simulink model "bh_compare_hand_MCKG_to_Ab"  (R2020b)
settings: Solver=ode23t  StartTime=0.0  StopTime=50  FixedStep=0.001  RelTol=1e-5  EnableMultiTasking=on
values from neighbouring files (symbols this model uses):
  K = [0.0865712753524 0.00277244570809 -0.0192153083791 -0.00162453351485 3.32348361895e-08 -1.41900444311e-08 -0.0932413563659 2.38058592401e-06 6.56188614095e-09 -0.0932413743514 2.52459639721e-09 9.53911962763e-08 ... (84 elements, 4x21)]    [CONFIRMED_bh_CONT_DES_RESULTS.mat]    (also in CONFIRMED_bh_CONT_DES_RESULTS_DISCRETE.mat = [-4.44584196463e-19 1.60298866655e-18 6.22915677006e-18 0 -9; CONFIRMED_bh_CONT_DES_RESULTS_DISCRETE_PRE_19a_using_DARE_SOLVER.mat = [-0.000193022438438 0.000285510081841 0.000531074046333 0.00; CONFIRMED_bh_CONT_DES_RESULTS_DISCRETE_R2019b.mat = [3.0073494701e-20 1.31173839205e-18 -5.80308139081e-19 0 8.7; CONFIRMED_bh_CONT_DES_RESULTS_PRE_19a_using_CARE_SOLVER.mat = [3.8473936011e-07 5.10337913269e-05 5.50269068807e-05 0.0072)
undefined symbols (not defined in the file or in its folder): P_elec, P_mot, P_one_prop, P_pend, P_veh, sigbuilder_block
libraries: simulink_extras x42, bh_6dof_LIBRARY x42, pid_lib x8, simulink x6
(part 1 of 3)
settings Model: Creator=bhorton  LastModifiedBy=bhorton
settings SolverCC: ZeroCrossAlgorithm=Adaptive
settings DataIOCC: SaveOutput=off  SignalLogging=off  DSMLogging=off  VisualizeSimOutput=off  SaveTime=off  ReturnWorkspaceOutputs=off
settings OptimizationCC: LifeSpan=inf
settings DebuggingCC: AllowSymbolicDim=off  PregeneratedLibrarySubsystemCodeDiagnostic=none  SFUnexpectedBacktrackingDiag=warning  SFNoUnconditionalDefaultTransitionDiag=warning  SFExecutionAtInitializationDiag=none  ArithmeticOperatorsInVariantConditions=warning
settings ModelReferenceCC: PropagateSignalLabelsOutOfModel=off
settings SFSimCC: SimUseLocalCustomCode=off  CustomCodeUndefinedFunction=UseInterfaceOnly
settings RTWCC: RTWUseLocalCustomCode=off
settings CodeAppCC: StateflowObjectComments=on
settings GRTTargetCC: TargetLangStandard=C89/C90 (ANSI)
settings ConfigComp: CovMetricSettings=dw  CovSaveCumulativeToWorkspaceVar=on  CovSaveSingleToWorkspaceVar=on  CovExternalEMLEnable=off
settings SimscapeCC: SimscapeNormalizeSystem=off
settings ExplorerConfigSet: InternalSimMechanicsExplorerSettings="<ExplorerConfiguration><canonicalview>default</canonicalview><AnimationSetting><BasePlaybackSpeed>1.0</BasePlaybackSpeed><PlaybackSpeedFactor>1.0</PlaybackSpeedFactor></AnimationSetting><TilePanel><TileInfo><Tiles Columns=\"2\" Count=\"4\" Rows=\"2\"><Column Weight=\"0.5\"/><Column Weight=\"0.5\"/><Row Weight=\"0.4994\"/><Row Weight=\"0.5006\"/><Tile Height=\"1\" Width=\"1\" X=\"0\" Y=\"0\"/><Tile Height=\"1\" Width=\"1\" X=\"0\" Y=\"1\"/><Tile Height=\"1\" Width=\"1\" X=\"1\" Y=\"0\"/><Tile Height=\"1\" Width=\"1\" X=\"1\" Y=\"1\"/></Tiles></TileInfo><SceneInfo><SceneViewer><BGColor><R>0.60000002384185791</R><G>0.60000002384185791</G><B>0.60000002384185791</B></BGColor><Camera><DoPerspective>off</DoPerspective><Position><X>0.108247136928821264</X><Y>-6.24186541247397919</Y><Z>0.0436626556988363723</Z></Position><Center><X>0.108247136928821264</X><Y>-0.000367992122906724006</Y><Z>0.0436626556988363723</Z></Center><Up><X>0</X><Y>-0</Y><Z>1</Z></Up><ViewLimDist>1</ViewLimDist><YLim>1.16644783469621482</YLim><XLim>1.16339430633313579</XLim></Camera></SceneViewer><SceneViewer><BGColor><R>0.60000002384185791</R><G>0.60000002384185791</G><B>0.60000002384185791</B></BGColor><Camera><DoPerspective>off</DoPerspective><Position><X>0.757932917509077875</X><Y>0.0622058730915643621</Y><Z>3.72898666655047251</Z></Position><Center><X>0.757932917509077875</X><Y>0.0622058730915643621</Y><Z>0.139377425336091543</Z></Center><Up><X>0</X><Y>1</Y><Z>-0</Z></Up><ViewLimDist>1</ViewLimDist><YLim>2.25856806031746737</YLim><XLim>2.2467739712296475</XLim></Camera></SceneViewer><SceneViewer><BGColor><R>0.60000002384185791</R><G>0.60000002384185791</G><B>0.60000002384185791</B></BGColor><Camera><DoPerspective>off</DoPerspective><Position><X>6.1954811663463758</X><Y>0.00989846582022124721</Y><Z>-0.0982778559424095921</Z></Position><Center><X>1.64798789726574491</X><Y>0.00989846582022124721</Y><Z>-0.0982778559424095921</Z></Center><Up><X>-0</X><Y>0</Y><Z>1</Z></Up><ViewLimDist>1</ViewLimDist><YLim>1.24345413764386392</YLim><XLim>1.24019902210029365</XLim></Camera></SceneViewer><SceneViewer><BGColor><R>0.60000002384185791</R><G>0.60000002384185791</G><B>0.60000002384185791</B></BGColor><Camera><DoPerspective>off</DoPerspective><Position><X>2.62526658870557483</X><Y>-2.63611357142327529</Y><Z>3.20950930741758134</Z></Position><Center><X>0.332369543668942558</X><Y>-0.343216526386576959</Y><Z>0.916612262380957166</Z></Center><Up><X>-0.408248290463863073</X><Y>0.408248290463863073</Y><Z>0.816496580927726145</Z></Up><ViewLimDist>1</ViewLimDist><YLim>1.98922512992447675</YLim><XLim>1.97883753133479279</XLim></Camera></SceneViewer></SceneInfo></TilePanel><MechEditorPanel><Cameras/><GfxPanelCameraMap/><VideoCreator><PlaybackSpeedRatio>1.0</PlaybackSpeedRatio><FrameRate>30</FrameRate><VideoFormat>Motion JPEG AVI</VideoFormat><FrameSize>auto</FrameSize></VideoCreator></MechEditorPanel></ExplorerConfiguration>"

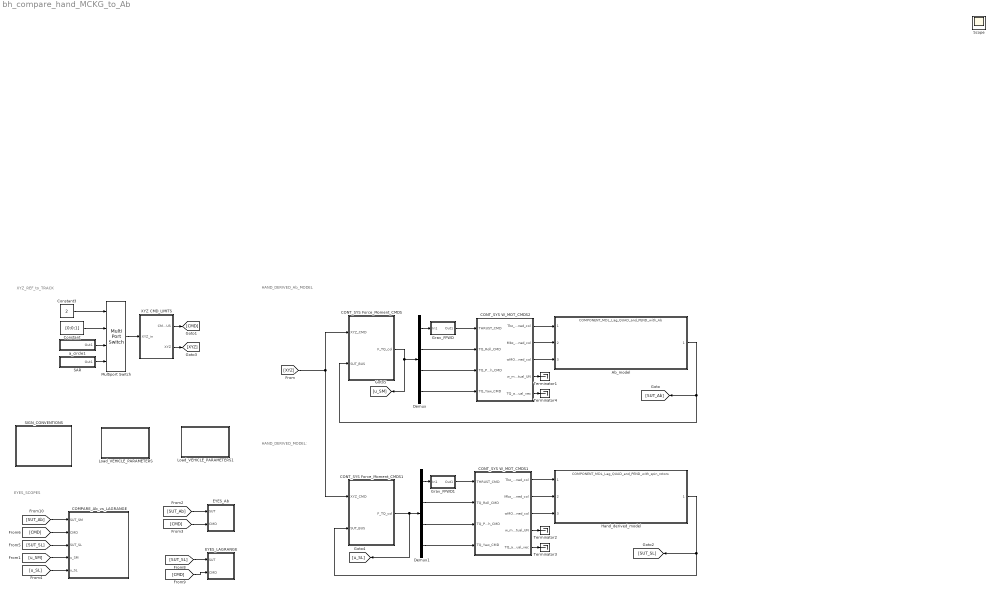
== system bh_compare_hand_MCKG_to_Ab ==
  note: XYZ_REF_to_TRACK
  note: EYES_SCOPES
  note: HAND_DERIVED_MODEL:
  note: HAND_DERIVED_Ab_MODEL
  Ab_model : ModelReference  ModelNameDialog=COMPONENT_MDL_Lag_QUAD_and_PEND_with_Ab.slx  SimulationMode=Normal  ModelReferenceVersion=2.3
  COMPARE_Ab_vs_LAGRANGE : Subsystem
  CONT_SYS Force_Moment_CMDS : Subsystem
  CONT_SYS Force_Moment_CMDS1 : Subsystem
  CONT_SYS W_MOT_CMDS1 : Subsystem
  CONT_SYS W_MOT_CMDS2 : Subsystem
  Constant : Constant  Value=[0;0;1]  VectorParams1D=off
  Constant3 : Constant  Value=2
  Demux : Demux
  Demux1 : Demux
  EYES_Ab : Subsystem
      mask Display: image('bh_PIC_SCOPE.jpg');
  EYES_LAGRANGE : Subsystem
      mask Display: image('bh_PIC_SCOPE.jpg');
  Grav_FFWD : Subsystem
  Grav_FFWD1 : Subsystem
  Hand_derived_model : ModelReference  ModelNameDialog=COMPONENT_MDL_Lag_QUAD_and_PEND_with_spin_rotors.slx  SimulationMode=Normal  ModelReferenceVersion=2.1
  Load_VEHICLE_PARAMETERS : Subsystem
      settings: OpenFcn=bh_create_local_params_QP
      mask Display: disp('Double click\nto\nLOAD\nvehicle and\n PENDULUM\n parameters')
  Load_VEHICLE_PARAMETERS1 : Subsystem
      settings: AttributesFormatString=OpenFcn = %<OpenFcn>  OpenFcn=load bh_CONT_DES_RESULTS.mat
      mask Display: disp('Double click\nto\nLOAD the\nControl LAW')
  Multiport Switch : MultiPortSwitch
  SAR : Subsystem
  SIGN_CONVENTIONS : Subsystem
  Terminator{1..4} (4 alike) : Terminator
  XYZ CMD_LIMITS : Subsystem
  a_circle1 : Subsystem
  Scope : Scope
  wires:
  [SUT_Ab] -> EYES_Ab/1(SUT)
  [CMD] -> EYES_Ab/2(CMD)
  Demux/1 -> Grav_FFWD/1(In1)
  Demux/2 -> CONT_SYS W_MOT_CMDS2/2(TQ_Roll_CMD)
  Demux/3 -> CONT_SYS W_MOT_CMDS2/3(TQ_Pitch_CMD)
  Demux/4 -> CONT_SYS W_MOT_CMDS2/4(TQ_Yaw_CMD)
  Grav_FFWD/1(Out1) -> CONT_SYS W_MOT_CMDS2/1(THRUST_CMD)
  Grav_FFWD1/1(Out1) -> CONT_SYS W_MOT_CMDS1/1(THRUST_CMD)
  Demux1/4 -> CONT_SYS W_MOT_CMDS1/4(TQ_Yaw_CMD)
  Demux1/2 -> CONT_SYS W_MOT_CMDS1/2(TQ_Roll_CMD)
  Demux1/3 -> CONT_SYS W_MOT_CMDS1/3(TQ_Pitch_CMD)
  CONT_SYS W_MOT_CMDS1/3(wMOT_signed_col) -> Hand_derived_model/3
  Demux1/1 -> Grav_FFWD1/1(In1)
  CONT_SYS W_MOT_CMDS1/5(TQ_actual_vec) -> Terminator3/1
  Hand_derived_model/1 -> [SUT_SL], CONT_SYS Force_Moment_CMDS1/2(SUT_BUS)
  CONT_SYS W_MOT_CMDS1/2(Mbz_signed_col) -> Hand_derived_model/2
  CONT_SYS W_MOT_CMDS1/4(w_mot_actual_UN) -> Terminator2/1
  [XYZ] -> CONT_SYS Force_Moment_CMDS/1(XYZ_CMD), CONT_SYS Force_Moment_CMDS1/1(XYZ_CMD)
  CONT_SYS W_MOT_CMDS1/1(Tbz_signed_col) -> Hand_derived_model/1
  CONT_SYS Force_Moment_CMDS/1(F_TQ_col) -> [u_SM], Demux/1
  CONT_SYS Force_Moment_CMDS1/1(F_TQ_col) -> [u_SL], Demux1/1
  [SUT_SL] -> COMPARE_Ab_vs_LAGRANGE/3(SUT_SL)
  [CMD] -> COMPARE_Ab_vs_LAGRANGE/2(CMD)
  [SUT_Ab] -> COMPARE_Ab_vs_LAGRANGE/1(SUT_SM)
  [u_SL] -> COMPARE_Ab_vs_LAGRANGE/5(u_SL)
  [u_SM] -> COMPARE_Ab_vs_LAGRANGE/4(u_SM)
  [SUT_SL] -> EYES_LAGRANGE/1(SUT)
  [CMD] -> EYES_LAGRANGE/2(CMD)
  a_circle1/1(Out1) -> Multiport Switch/3
  Constant/1 -> Multiport Switch/2
  SAR/1(Out1) -> Multiport Switch/4
  Constant3/1 -> Multiport Switch/1
  Multiport Switch/1 -> XYZ CMD_LIMITS/1(XYZ_in)
  XYZ CMD_LIMITS/1(CMD_BUS) -> [CMD]
  XYZ CMD_LIMITS/2(XYZ) -> [XYZ]
  CONT_SYS W_MOT_CMDS2/1(Tbz_signed_col) -> Ab_model/1
  CONT_SYS W_MOT_CMDS2/2(Mbz_signed_col) -> Ab_model/2
  CONT_SYS W_MOT_CMDS2/3(wMOT_signed_col) -> Ab_model/3
  Ab_model/1 -> [SUT_Ab], CONT_SYS Force_Moment_CMDS/2(SUT_BUS)
  CONT_SYS W_MOT_CMDS2/4(w_mot_actual_UN) -> Terminator1/1
  CONT_SYS W_MOT_CMDS2/5(TQ_actual_vec) -> Terminator4/1

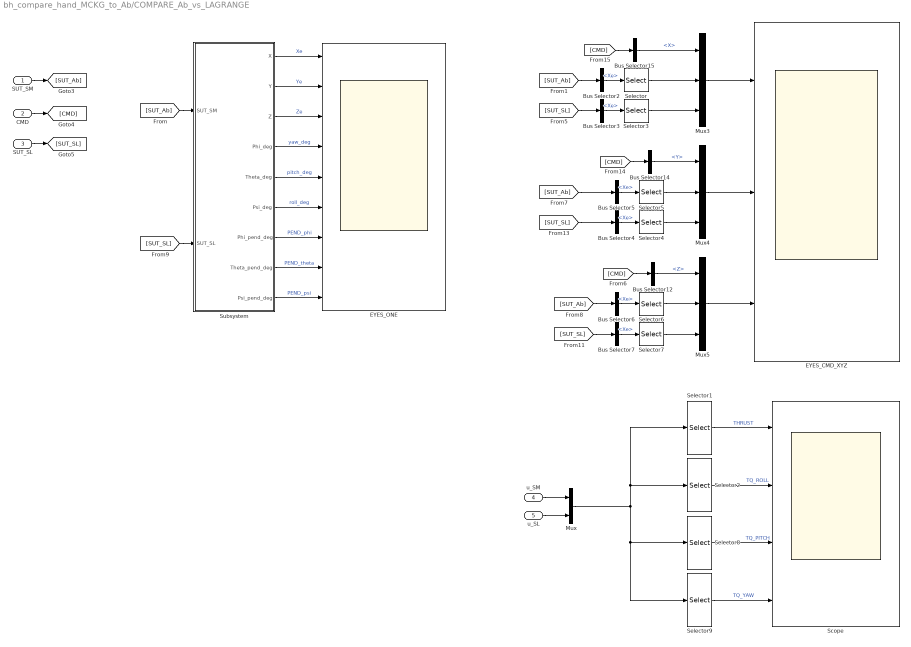
== system bh_compare_hand_MCKG_to_Ab/COMPARE_Ab_vs_LAGRANGE ==
  SUT_SM : Inport
  CMD : Inport  Port=2
  SUT_SL : Inport  Port=3
  u_SM : Inport  Port=4
  u_SL : Inport  Port=5
  Bus Selector12 : BusSelector  OutputSignals=Z
  Bus Selector14 : BusSelector  OutputSignals=Y
  Bus Selector15 : BusSelector  OutputSignals=X
  Bus Selector{2..7} (6 alike) : BusSelector  OutputSignals=Xe
  EYES_CMD_XYZ : Scope  NumInputPorts=3
  EYES_ONE : Scope  NumInputPorts=9
  Mux : Mux  Inputs=2
  Mux3 : Mux  Inputs=3
  Mux4 : Mux  Inputs=3
  Mux5 : Mux  Inputs=3
  Scope : Scope  NumInputPorts=4
  Selector : Selector  InputPortWidth=3  IndexOptions=Index vector (dialog)  Indices=1  OutputSizes=1
  Selector1 : Selector  InputPortWidth=8  IndexOptions=Index vector (dialog)  Indices=[1 5]  OutputSizes=1
  Selector2 : Selector  InputPortWidth=8  IndexOptions=Index vector (dialog)  Indices=[2 6]  OutputSizes=1
  Selector3 : Selector  InputPortWidth=3  IndexOptions=Index vector (dialog)  Indices=1  OutputSizes=1
  Selector4 : Selector  InputPortWidth=3  IndexOptions=Index vector (dialog)  Indices=2  OutputSizes=1
  Selector5 : Selector  InputPortWidth=3  IndexOptions=Index vector (dialog)  Indices=2  OutputSizes=1
  Selector6 : Selector  InputPortWidth=3  IndexOptions=Index vector (dialog)  Indices=3  OutputSizes=1
  Selector7 : Selector  InputPortWidth=3  IndexOptions=Index vector (dialog)  Indices=3  OutputSizes=1
  Selector8 : Selector  InputPortWidth=8  IndexOptions=Index vector (dialog)  Indices=[3 7]  OutputSizes=1
  Selector9 : Selector  InputPortWidth=8  IndexOptions=Index vector (dialog)  Indices=[4 8]  OutputSizes=1
  Subsystem : Subsystem
  wires:
  Subsystem/9(Psi_pend_deg) -> EYES_ONE/9  "PEND_psi"
  Subsystem/1(X) -> EYES_ONE/1  "Xe"
  Subsystem/8(Theta_pend_deg) -> EYES_ONE/8  "PEND_theta"
  Subsystem/4(Phi_deg) -> EYES_ONE/4  "yaw_deg"
  Subsystem/6(Psi_deg) -> EYES_ONE/6  "roll_deg"
  Subsystem/5(Theta_deg) -> EYES_ONE/5  "pitch_deg"
  Subsystem/2(Y) -> EYES_ONE/2  "Ye"
  Subsystem/3(Z) -> EYES_ONE/3  "Ze"
  Subsystem/7(Phi_pend_deg) -> EYES_ONE/7  "PEND_phi"
  SUT_SM/1 -> [SUT_Ab]
  CMD/1 -> [CMD]
  SUT_SL/1 -> [SUT_SL]
  Mux4/1 -> EYES_CMD_XYZ/2
  Mux3/1 -> EYES_CMD_XYZ/1
  [SUT_Ab] -> Bus Selector2/1
  Bus Selector2/1 -> Selector/1  "<Xe>"
  Bus Selector3/1 -> Selector3/1  "<Xe>"
  [SUT_SL] -> Bus Selector3/1
  Bus Selector4/1 -> Selector4/1  "<Xe>"
  [SUT_SL] -> Bus Selector4/1
  [SUT_Ab] -> Bus Selector5/1
  Bus Selector5/1 -> Selector5/1  "<Xe>"
  Selector4/1 -> Mux4/3
  Selector5/1 -> Mux4/2
  [SUT_Ab] -> Bus Selector6/1
  Bus Selector6/1 -> Selector6/1  "<Xe>"
  Bus Selector7/1 -> Selector7/1  "<Xe>"
  [SUT_SL] -> Bus Selector7/1
  Selector7/1 -> Mux5/3
  Selector6/1 -> Mux5/2
  [CMD] -> Bus Selector12/1
  Bus Selector12/1 -> Mux5/1  "<Z>"
  Bus Selector14/1 -> Mux4/1  "<Y>"
  [CMD] -> Bus Selector14/1
  [CMD] -> Bus Selector15/1
  Bus Selector15/1 -> Mux3/1  "<X>"
  Selector/1 -> Mux3/2
  Selector3/1 -> Mux3/3
  Mux5/1 -> EYES_CMD_XYZ/3
  [SUT_Ab] -> Subsystem/1(SUT_SM)
  [SUT_SL] -> Subsystem/2(SUT_SL)
  u_SL/1 -> Mux/2
  u_SM/1 -> Mux/1
  Selector1/1 -> Scope/1  "THRUST"
  Selector2/1 -> Scope/2  "TQ_ROLL"
  Selector8/1 -> Scope/3  "TQ_PITCH"
  Selector9/1 -> Scope/4  "TQ_YAW"
  Mux/1 -> Selector9/1, Selector8/1, Selector1/1, Selector2/1

== system bh_compare_hand_MCKG_to_Ab/CONT_SYS Force_Moment_CMDS ==
  XYZ_CMD : Inport
  SUT_BUS : Inport  Port=2
  Bus Selector : BusSelector  OutputSignals=Xe
  Bus Selector1 : BusSelector  OutputSignals=DOT_phi_theta_psi,Ve,pend_bus.DOT_phi_theta_psi,phi_theta_psi,Xe,pend_bus.phi_theta_psi
  Constant1 : Constant  Value=[0;0;0]  VectorParams1D=off
  Constant2 : Constant  Value=K  VectorParams1D=off
  Gain1 : Gain  Gain=-1
  Integrator : Integrator  InitialConditionSource=external
  Mux : Mux  Inputs=7
  Product1 : Product  Multiplication=Matrix(*)
  Reshape{,1..7} (8 alike) : Reshape  OutputDimensionality=Column vector (2-D)
  Sum : Sum  Inputs=|+-
  F_TQ_col : Outport  VectorParamsAs1DForOutWhenUnconnected=off
  wires:
  SUT_BUS/1 -> [SUT], Bus Selector/1
  Constant1/1 -> Integrator/2
  Integrator/1 -> Reshape/1
  Reshape/1 -> Mux/7
  XYZ_CMD/1 -> Sum/1
  Sum/1 -> Integrator/1
  Bus Selector/1 -> Sum/2  "<Xe>"
  [SUT] -> Bus Selector1/1
  Bus Selector1/1 -> Reshape1/1  "<DOT_phi_theta_psi>"
  Bus Selector1/2 -> Reshape2/1  "<Ve>"
  Bus Selector1/4 -> Reshape3/1  "<phi_theta_psi>"
  Bus Selector1/5 -> Reshape4/1  "<Xe>"
  Constant2/1 -> Gain1/1
  Gain1/1 -> Product1/1
  Mux/1 -> Product1/2
  Product1/1 -> Reshape5/1
  Reshape5/1 -> F_TQ_col/1
  Bus Selector1/6 -> Reshape6/1  "<phi_theta_psi>"
  Bus Selector1/3 -> Reshape7/1  "<DOT_phi_theta_psi>"
  Reshape1/1 -> Mux/1
  Reshape2/1 -> Mux/2
  Reshape7/1 -> Mux/3
  Reshape3/1 -> Mux/4
  Reshape4/1 -> Mux/5
  Reshape6/1 -> Mux/6

== system bh_compare_hand_MCKG_to_Ab/CONT_SYS Force_Moment_CMDS1 ==
  XYZ_CMD : Inport
  SUT_BUS : Inport  Port=2
  Bus Selector : BusSelector  OutputSignals=Xe
  Bus Selector1 : BusSelector  OutputSignals=DOT_phi_theta_psi,Ve,pend_bus.DOT_phi_theta_psi,phi_theta_psi,Xe,pend_bus.phi_theta_psi
  Constant1 : Constant  Value=[0;0;0]  VectorParams1D=off
  Constant2 : Constant  Value=K  VectorParams1D=off
  Constant3 : Constant  Value=P_veh.mass
  Gain : Gain  Gain=9.81
  Gain1 : Gain  Gain=-1
  Integrator : Integrator  InitialConditionSource=external
  Mux : Mux  Inputs=7
  Product1 : Product  Multiplication=Matrix(*)
  Reshape{,1..7} (8 alike) : Reshape  OutputDimensionality=Column vector (2-D)
  Sum : Sum  Inputs=|+-
  F_TQ_col : Outport  VectorParamsAs1DForOutWhenUnconnected=off
  wires:
  SUT_BUS/1 -> [SUT], Bus Selector/1
  Constant3/1 -> Gain/1
  Constant1/1 -> Integrator/2
  Integrator/1 -> Reshape/1
  Reshape/1 -> Mux/7
  XYZ_CMD/1 -> Sum/1
  Sum/1 -> Integrator/1
  Bus Selector/1 -> Sum/2  "<Xe>"
  [SUT] -> Bus Selector1/1
  Bus Selector1/1 -> Reshape1/1  "<DOT_phi_theta_psi>"
  Bus Selector1/2 -> Reshape2/1  "<Ve>"
  Bus Selector1/4 -> Reshape3/1  "<phi_theta_psi>"
  Bus Selector1/5 -> Reshape4/1  "<Xe>"
  Constant2/1 -> Gain1/1
  Gain1/1 -> Product1/1
  Mux/1 -> Product1/2
  Product1/1 -> Reshape5/1
  Reshape5/1 -> F_TQ_col/1
  Bus Selector1/6 -> Reshape6/1  "<phi_theta_psi>"
  Bus Selector1/3 -> Reshape7/1  "<DOT_phi_theta_psi>"
  Reshape1/1 -> Mux/1
  Reshape2/1 -> Mux/2
  Reshape7/1 -> Mux/3
  Reshape3/1 -> Mux/4
  Reshape4/1 -> Mux/5
  Reshape6/1 -> Mux/6

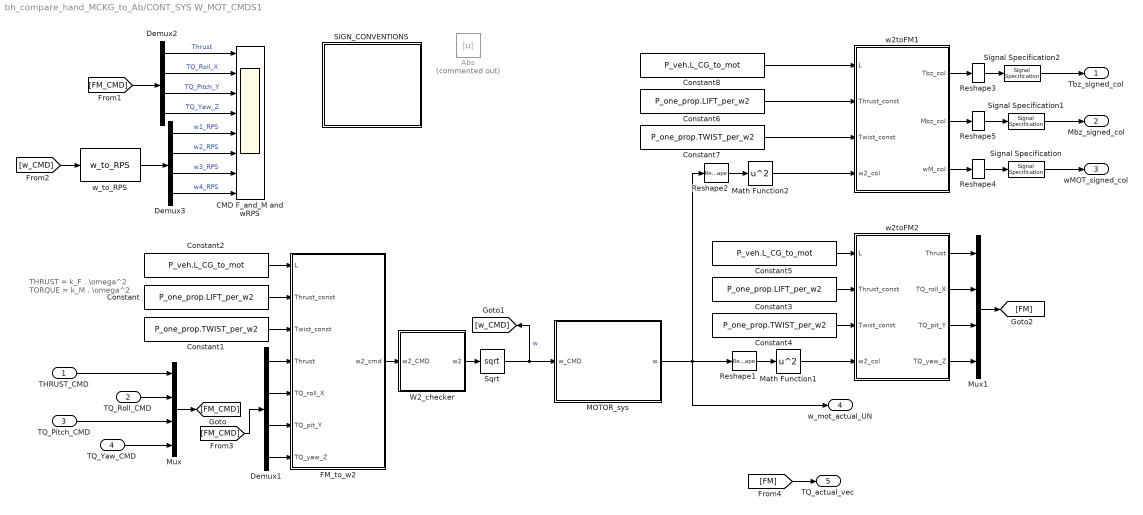
== system bh_compare_hand_MCKG_to_Ab/CONT_SYS W_MOT_CMDS1 ==
  note: THRUST = k_F . \omega^2
      |
      | TORQUE = k_M . \omega^2
  THRUST_CMD : Inport
  TQ_Roll_CMD : Inport  Port=2
  TQ_Pitch_CMD : Inport  Port=3
  TQ_Yaw_CMD : Inport  Port=4
  Abs : Abs  Commented=on
  CMD F_and_M and wRPS : Scope  NumInputPorts=8
  Constant : Constant  Value=P_one_prop.LIFT_per_w2
  Constant1 : Constant  Value=P_one_prop.TWIST_per_w2
  Constant2 : Constant  Value=P_veh.L_CG_to_mot
  Constant3 : Constant  Value=P_one_prop.LIFT_per_w2
  Constant4 : Constant  Value=P_one_prop.TWIST_per_w2
  Constant5 : Constant  Value=P_veh.L_CG_to_mot
  Constant6 : Constant  Value=P_one_prop.LIFT_per_w2
  Constant7 : Constant  Value=P_one_prop.TWIST_per_w2
  Constant8 : Constant  Value=P_veh.L_CG_to_mot
  Demux1 : Demux
  Demux2 : Demux
  Demux3 : Demux
  FM_to_w2 : MATLAB Function  TreatAsAtomicUnit=on
  MOTOR_sys : Subsystem
      mask Display: image('bh_PIC_MOTOR.jpg');
  Math Function1 : Math  Operator=square  SignedPower=on  SaturateOnIntegerOverflow=on
  Math Function2 : Math  Operator=square  SignedPower=on  SaturateOnIntegerOverflow=on
  Mux : Mux
  Mux1 : Mux
  Reshape{1..5} (5 alike) : Reshape  OutputDimensionality=Column vector (2-D)
  SIGN_CONVENTIONS : Subsystem
  Signal Specification : SignalSpecification  Dimensions=[4,1]
  Signal Specification1 : SignalSpecification  Dimensions=[4,1]
  Signal Specification2 : SignalSpecification  Dimensions=[4,1]
  Sqrt : Sqrt  SaturateOnIntegerOverflow=on
  W2_checker : Subsystem
  w2toFM1 : MATLAB Function  TreatAsAtomicUnit=on
  w2toFM2 : MATLAB Function  TreatAsAtomicUnit=on
  w_to_RPS : bh_6dof_LIBRARY/MODELS/w_to_RPS  SystemSampleTime=-1  VariantActivationTime=update diagram  Latency=0  AutoFrameSizeCalculation=off
  Tbz_signed_col : Outport  VectorParamsAs1DForOutWhenUnconnected=off
  Mbz_signed_col : Outport  Port=2  VectorParamsAs1DForOutWhenUnconnected=off
  wMOT_signed_col : Outport  Port=3  VectorParamsAs1DForOutWhenUnconnected=off
  w_mot_actual_UN : Outport  Port=4  VectorParamsAs1DForOutWhenUnconnected=off
  TQ_actual_vec : Outport  Port=5  VectorParamsAs1DForOutWhenUnconnected=off
  wires:
  Constant1/1 -> FM_to_w2/3(Twist_const)
  Constant/1 -> FM_to_w2/2(Thrust_const)
  Constant2/1 -> FM_to_w2/1(L)
  Sqrt/1 -> MOTOR_sys/1(w_CMD), [w_CMD]  "w"
  W2_checker/1(w2) -> Sqrt/1
  Demux1/1 -> FM_to_w2/4(Thrust)
  Demux1/2 -> FM_to_w2/5(TQ_roll_X)
  Demux1/3 -> FM_to_w2/6(TQ_pit_Y)
  Demux1/4 -> FM_to_w2/7(TQ_yaw_Z)
  THRUST_CMD/1 -> Mux/1
  TQ_Roll_CMD/1 -> Mux/2
  TQ_Pitch_CMD/1 -> Mux/3
  TQ_Yaw_CMD/1 -> Mux/4
  Mux/1 -> [FM_CMD]
  [FM_CMD] -> Demux1/1
  Demux2/1 -> CMD F_and_M and wRPS/1  "Thrust"
  Demux2/2 -> CMD F_and_M and wRPS/2  "TQ_Roll_X"
  Demux2/3 -> CMD F_and_M and wRPS/3  "TQ_Pitch_Y"
  Demux2/4 -> CMD F_and_M and wRPS/4  "TQ_Yaw_Z"
  Demux3/2 -> CMD F_and_M and wRPS/6  "w2_RPS"
  Demux3/1 -> CMD F_and_M and wRPS/5  "w1_RPS"
  Demux3/4 -> CMD F_and_M and wRPS/8  "w4_RPS"
  Demux3/3 -> CMD F_and_M and wRPS/7  "w3_RPS"
  [FM_CMD] -> Demux2/1
  w_to_RPS/1 -> Demux3/1
  [w_CMD] -> w_to_RPS/1
  Constant3/1 -> w2toFM2/2(Thrust_const)
  Constant4/1 -> w2toFM2/3(Twist_const)
  Constant5/1 -> w2toFM2/1(L)
  Mux1/1 -> [FM]
  Reshape1/1 -> Math Function1/1
  Math Function1/1 -> w2toFM2/4(w2_col)
  [FM] -> TQ_actual_vec/1
  w2toFM2/1(Thrust) -> Mux1/1
  w2toFM2/2(TQ_roll_X) -> Mux1/2
  w2toFM2/3(TQ_pit_Y) -> Mux1/3
  w2toFM2/4(TQ_yaw_Z) -> Mux1/4
  Reshape2/1 -> Math Function2/1
  Math Function2/1 -> w2toFM1/4(w2_col)
  Constant7/1 -> w2toFM1/3(Twist_const)
  Constant6/1 -> w2toFM1/2(Thrust_const)
  Constant8/1 -> w2toFM1/1(L)
  w2toFM1/2(Mbz_col) -> Reshape5/1
  w2toFM1/1(Tbz_col) -> Reshape3/1
  w2toFM1/3(wM_col) -> Reshape4/1
  Reshape3/1 -> Signal Specification2/1
  Reshape5/1 -> Signal Specification1/1
  Reshape4/1 -> Signal Specification/1
  Signal Specification2/1 -> Tbz_signed_col/1
  Signal Specification1/1 -> Mbz_signed_col/1
  Signal Specification/1 -> wMOT_signed_col/1
  FM_to_w2/1(w2_cmd) -> W2_checker/1(w2_CMD)
  MOTOR_sys/1(w) -> Reshape1/1, w_mot_actual_UN/1, Reshape2/1

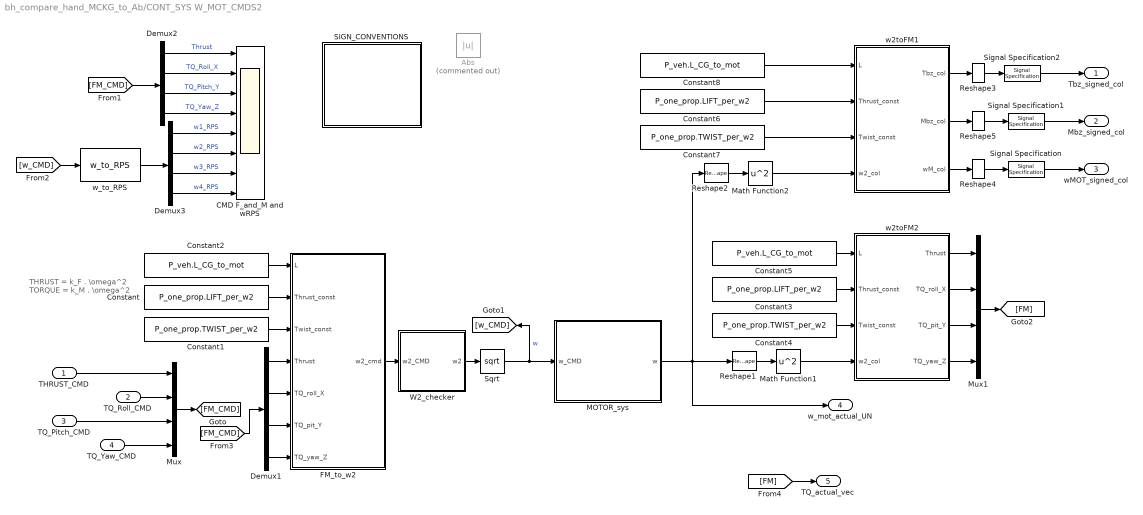
== system bh_compare_hand_MCKG_to_Ab/CONT_SYS W_MOT_CMDS2 ==
  note: THRUST = k_F . \omega^2
      |
      | TORQUE = k_M . \omega^2
  THRUST_CMD : Inport
  TQ_Roll_CMD : Inport  Port=2
  TQ_Pitch_CMD : Inport  Port=3
  TQ_Yaw_CMD : Inport  Port=4
  Abs : Abs  Commented=on
  CMD F_and_M and wRPS : Scope  NumInputPorts=8
  Constant : Constant  Value=P_one_prop.LIFT_per_w2
  Constant1 : Constant  Value=P_one_prop.TWIST_per_w2
  Constant2 : Constant  Value=P_veh.L_CG_to_mot
  Constant3 : Constant  Value=P_one_prop.LIFT_per_w2
  Constant4 : Constant  Value=P_one_prop.TWIST_per_w2
  Constant5 : Constant  Value=P_veh.L_CG_to_mot
  Constant6 : Constant  Value=P_one_prop.LIFT_per_w2
  Constant7 : Constant  Value=P_one_prop.TWIST_per_w2
  Constant8 : Constant  Value=P_veh.L_CG_to_mot
  Demux1 : Demux
  Demux2 : Demux
  Demux3 : Demux
  FM_to_w2 : MATLAB Function  TreatAsAtomicUnit=on
  MOTOR_sys : Subsystem
      mask Display: image('bh_PIC_MOTOR.jpg');
  Math Function1 : Math  Operator=square  SignedPower=on  SaturateOnIntegerOverflow=on
  Math Function2 : Math  Operator=square  SignedPower=on  SaturateOnIntegerOverflow=on
  Mux : Mux
  Mux1 : Mux
  Reshape{1..5} (5 alike) : Reshape  OutputDimensionality=Column vector (2-D)
  SIGN_CONVENTIONS : Subsystem
  Signal Specification : SignalSpecification  Dimensions=[4,1]
  Signal Specification1 : SignalSpecification  Dimensions=[4,1]
  Signal Specification2 : SignalSpecification  Dimensions=[4,1]
  Sqrt : Sqrt  SaturateOnIntegerOverflow=on
  W2_checker : Subsystem
  w2toFM1 : MATLAB Function  TreatAsAtomicUnit=on
  w2toFM2 : MATLAB Function  TreatAsAtomicUnit=on
  w_to_RPS : bh_6dof_LIBRARY/MODELS/w_to_RPS  SystemSampleTime=-1  VariantActivationTime=update diagram  Latency=0  AutoFrameSizeCalculation=off
  Tbz_signed_col : Outport  VectorParamsAs1DForOutWhenUnconnected=off
  Mbz_signed_col : Outport  Port=2  VectorParamsAs1DForOutWhenUnconnected=off
  wMOT_signed_col : Outport  Port=3  VectorParamsAs1DForOutWhenUnconnected=off
  w_mot_actual_UN : Outport  Port=4  VectorParamsAs1DForOutWhenUnconnected=off
  TQ_actual_vec : Outport  Port=5  VectorParamsAs1DForOutWhenUnconnected=off
  wires:
  Constant1/1 -> FM_to_w2/3(Twist_const)
  Constant/1 -> FM_to_w2/2(Thrust_const)
  Constant2/1 -> FM_to_w2/1(L)
  Sqrt/1 -> MOTOR_sys/1(w_CMD), [w_CMD]  "w"
  W2_checker/1(w2) -> Sqrt/1
  Demux1/1 -> FM_to_w2/4(Thrust)
  Demux1/2 -> FM_to_w2/5(TQ_roll_X)
  Demux1/3 -> FM_to_w2/6(TQ_pit_Y)
  Demux1/4 -> FM_to_w2/7(TQ_yaw_Z)
  THRUST_CMD/1 -> Mux/1
  TQ_Roll_CMD/1 -> Mux/2
  TQ_Pitch_CMD/1 -> Mux/3
  TQ_Yaw_CMD/1 -> Mux/4
  Mux/1 -> [FM_CMD]
  [FM_CMD] -> Demux1/1
  Demux2/1 -> CMD F_and_M and wRPS/1  "Thrust"
  Demux2/2 -> CMD F_and_M and wRPS/2  "TQ_Roll_X"
  Demux2/3 -> CMD F_and_M and wRPS/3  "TQ_Pitch_Y"
  Demux2/4 -> CMD F_and_M and wRPS/4  "TQ_Yaw_Z"
  Demux3/2 -> CMD F_and_M and wRPS/6  "w2_RPS"
  Demux3/1 -> CMD F_and_M and wRPS/5  "w1_RPS"
  Demux3/4 -> CMD F_and_M and wRPS/8  "w4_RPS"
  Demux3/3 -> CMD F_and_M and wRPS/7  "w3_RPS"
  [FM_CMD] -> Demux2/1
  w_to_RPS/1 -> Demux3/1
  [w_CMD] -> w_to_RPS/1
  Constant3/1 -> w2toFM2/2(Thrust_const)
  Constant4/1 -> w2toFM2/3(Twist_const)
  Constant5/1 -> w2toFM2/1(L)
  Mux1/1 -> [FM]
  Reshape1/1 -> Math Function1/1
  Math Function1/1 -> w2toFM2/4(w2_col)
  [FM] -> TQ_actual_vec/1
  w2toFM2/1(Thrust) -> Mux1/1
  w2toFM2/2(TQ_roll_X) -> Mux1/2
  w2toFM2/3(TQ_pit_Y) -> Mux1/3
  w2toFM2/4(TQ_yaw_Z) -> Mux1/4
  Reshape2/1 -> Math Function2/1
  Math Function2/1 -> w2toFM1/4(w2_col)
  Constant7/1 -> w2toFM1/3(Twist_const)
  Constant6/1 -> w2toFM1/2(Thrust_const)
  Constant8/1 -> w2toFM1/1(L)
  w2toFM1/2(Mbz_col) -> Reshape5/1
  w2toFM1/1(Tbz_col) -> Reshape3/1
  w2toFM1/3(wM_col) -> Reshape4/1
  Reshape3/1 -> Signal Specification2/1
  Reshape5/1 -> Signal Specification1/1
  Reshape4/1 -> Signal Specification/1
  Signal Specification2/1 -> Tbz_signed_col/1
  Signal Specification1/1 -> Mbz_signed_col/1
  Signal Specification/1 -> wMOT_signed_col/1
  FM_to_w2/1(w2_cmd) -> W2_checker/1(w2_CMD)
  MOTOR_sys/1(w) -> Reshape1/1, w_mot_actual_UN/1, Reshape2/1

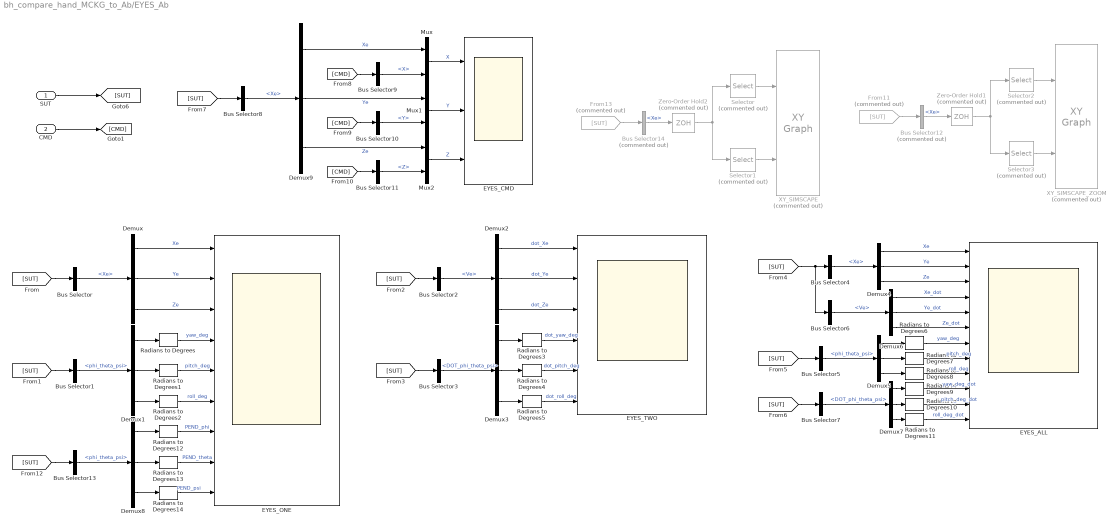
== system bh_compare_hand_MCKG_to_Ab/EYES_Ab ==
  SUT : Inport
  CMD : Inport  Port=2
  Bus Selector : BusSelector  OutputSignals=Xe
  Bus Selector1 : BusSelector  OutputSignals=phi_theta_psi
  Bus Selector10 : BusSelector  OutputSignals=Y
  Bus Selector11 : BusSelector  OutputSignals=Z
  Bus Selector12 : BusSelector  Commented=on  OutputSignals=Xe
  Bus Selector13 : BusSelector  OutputSignals=pend_bus.phi_theta_psi
  Bus Selector14 : BusSelector  Commented=on  OutputSignals=Xe
  Bus Selector2 : BusSelector  OutputSignals=Ve
  Bus Selector3 : BusSelector  OutputSignals=DOT_phi_theta_psi
  Bus Selector4 : BusSelector  OutputSignals=Xe
  Bus Selector5 : BusSelector  OutputSignals=phi_theta_psi
  Bus Selector6 : BusSelector  OutputSignals=Ve
  Bus Selector7 : BusSelector  OutputSignals=DOT_phi_theta_psi
  Bus Selector8 : BusSelector  OutputSignals=Xe
  Bus Selector9 : BusSelector  OutputSignals=X
  Demux{,1..9} (10 alike) : Demux  Outputs=3
  EYES_ALL : Scope  NumInputPorts=12
  EYES_CMD : Scope  NumInputPorts=3
  EYES_ONE : Scope  NumInputPorts=9
  EYES_TWO : Scope  NumInputPorts=6
  From11 : From  Commented=on  GotoTag=SUT
  From13 : From  Commented=on  GotoTag=SUT
  Mux : Mux  Inputs=2
  Mux1 : Mux  Inputs=2
  Mux2 : Mux  Inputs=2
  Radians to Degrees{,1..14} (15 alike) : simulink_extras/Transformations/Radians to Degrees
  Selector : Selector  Commented=on  InputPortWidth=3  IndexOptions=Index vector (dialog)  Indices=1  OutputSizes=1
  Selector1 : Selector  Commented=on  InputPortWidth=3  IndexOptions=Index vector (dialog)  Indices=2  OutputSizes=1
  Selector2 : Selector  Commented=on  InputPortWidth=3  IndexOptions=Index vector (dialog)  Indices=1  OutputSizes=1
  Selector3 : Selector  Commented=on  InputPortWidth=3  IndexOptions=Index vector (dialog)  Indices=2  OutputSizes=1
  XY_SIMSCAPE : simulink/Sinks/XY Graph  Commented=on  xmin=-1  xmax=30  ymin=-1  ymax=35  st=-1
  XY_SIMSCAPE_ZOOM : simulink/Sinks/XY Graph  Commented=on  xmin=-3  xmax=3  ymin=-3  ymax=3  st=-1
  Zero-Order Hold1 : ZeroOrderHold  Commented=on  SampleTime=0.1
  Zero-Order Hold2 : ZeroOrderHold  Commented=on  SampleTime=0.1
  wires:
  SUT/1 -> [SUT]
  [SUT] -> Bus Selector/1
  Demux/2 -> EYES_ONE/2  "Ye"
  Demux/3 -> EYES_ONE/3  "Ze"
  Demux/1 -> EYES_ONE/1  "Xe"
  Bus Selector/1 -> Demux/1  "<Xe>"
  Bus Selector1/1 -> Demux1/1  "<phi_theta_psi>"
  [SUT] -> Bus Selector1/1
  Demux1/1 -> Radians to Degrees/1
  Radians to Degrees/1 -> EYES_ONE/4  "yaw_deg"
  Radians to Degrees1/1 -> EYES_ONE/5  "pitch_deg"
  Radians to Degrees2/1 -> EYES_ONE/6  "roll_deg"
  Demux1/3 -> Radians to Degrees2/1
  Demux1/2 -> Radians to Degrees1/1
  [SUT] -> Bus Selector2/1
  Demux2/2 -> EYES_TWO/2  "dot_Ye"
  Demux2/3 -> EYES_TWO/3  "dot_Ze"
  Demux2/1 -> EYES_TWO/1  "dot_Xe"
  Bus Selector2/1 -> Demux2/1  "<Ve>"
  Bus Selector3/1 -> Demux3/1  "<DOT_phi_theta_psi>"
  [SUT] -> Bus Selector3/1
  Demux3/1 -> Radians to Degrees3/1
  Radians to Degrees3/1 -> EYES_TWO/4  "dot_yaw_deg"
  Radians to Degrees4/1 -> EYES_TWO/5  "dot_pitch_deg"
  Radians to Degrees5/1 -> EYES_TWO/6  "dot_roll_deg"
  Demux3/3 -> Radians to Degrees5/1
  Demux3/2 -> Radians to Degrees4/1
  [SUT] -> Bus Selector6/1, Bus Selector4/1
  Demux4/2 -> EYES_ALL/2  "Ye"
  Demux4/3 -> EYES_ALL/3  "Ze"
  Demux4/1 -> EYES_ALL/1  "Xe"
  Bus Selector4/1 -> Demux4/1  "<Xe>"
  Bus Selector5/1 -> Demux5/1  "<phi_theta_psi>"
  [SUT] -> Bus Selector5/1
  Demux5/1 -> Radians to Degrees6/1
  Demux6/1 -> EYES_ALL/4  "Xe_dot"
  Demux6/2 -> EYES_ALL/5  "Ye_dot"
  Demux6/3 -> EYES_ALL/6  "Ze_dot"
  Demux5/3 -> Radians to Degrees8/1
  Demux5/2 -> Radians to Degrees7/1
  Bus Selector6/1 -> Demux6/1  "<Ve>"
  Radians to Degrees6/1 -> EYES_ALL/7  "yaw_deg"
  Radians to Degrees7/1 -> EYES_ALL/8  "pitch_deg"
  Radians to Degrees8/1 -> EYES_ALL/9  "roll_deg"
  Bus Selector7/1 -> Demux7/1  "<DOT_phi_theta_psi>"
  [SUT] -> Bus Selector7/1
  Demux7/1 -> Radians to Degrees9/1
  Demux7/2 -> Radians to Degrees10/1
  Demux7/3 -> Radians to Degrees11/1
  Radians to Degrees9/1 -> EYES_ALL/10  "yaw_deg_dot"
  Radians to Degrees10/1 -> EYES_ALL/11  "pitch_deg_dot"
  Radians to Degrees11/1 -> EYES_ALL/12  "roll_deg_dot"
  CMD/1 -> [CMD]
  [SUT] -> Bus Selector8/1
  Demux9/2 -> Mux1/1  "Ye"
  Demux9/1 -> Mux/1  "Xe"
  Bus Selector8/1 -> Demux9/1  "<Xe>"
  Mux/1 -> EYES_CMD/1  "X"
  Mux1/1 -> EYES_CMD/2  "Y"
  Mux2/1 -> EYES_CMD/3  "Z"
  Demux9/3 -> Mux2/1  "Ze"
  [CMD] -> Bus Selector9/1
  Bus Selector9/1 -> Mux/2  "<X>"
  [CMD] -> Bus Selector10/1
  Bus Selector10/1 -> Mux1/2  "<Y>"
  [CMD] -> Bus Selector11/1
  Bus Selector11/1 -> Mux2/2  "<Z>"
  From13/1 -> Bus Selector14/1
  Bus Selector14/1 -> Zero-Order Hold2/1  "<Xe>"
  Zero-Order Hold2/1 -> Selector1/1, Selector/1
  Selector1/1 -> XY_SIMSCAPE/2
  Selector/1 -> XY_SIMSCAPE/1
  [SUT] -> Bus Selector13/1
  Bus Selector13/1 -> Demux8/1  "<phi_theta_psi>"
  Demux8/3 -> Radians to Degrees14/1
  Demux8/2 -> Radians to Degrees13/1
  Demux8/1 -> Radians to Degrees12/1
  Radians to Degrees12/1 -> EYES_ONE/7  "PEND_phi"
  Radians to Degrees13/1 -> EYES_ONE/8  "PEND_theta"
  Radians to Degrees14/1 -> EYES_ONE/9  "PEND_psi"
  From11/1 -> Bus Selector12/1
  Selector3/1 -> XY_SIMSCAPE_ZOOM/2
  Bus Selector12/1 -> Zero-Order Hold1/1  "<Xe>"
  Zero-Order Hold1/1 -> Selector3/1, Selector2/1
  Selector2/1 -> XY_SIMSCAPE_ZOOM/1

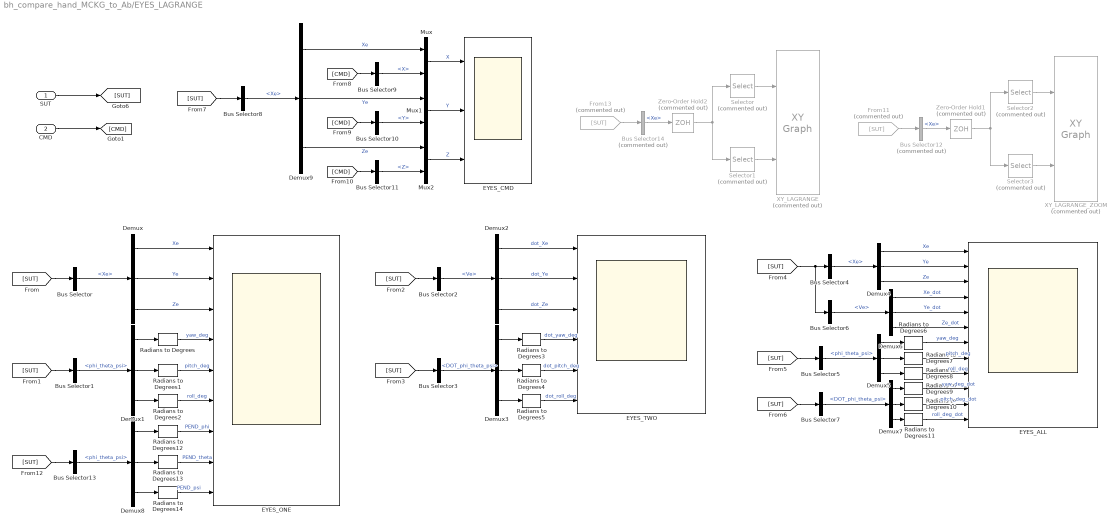
== system bh_compare_hand_MCKG_to_Ab/EYES_LAGRANGE ==
  SUT : Inport
  CMD : Inport  Port=2
  Bus Selector : BusSelector  OutputSignals=Xe
  Bus Selector1 : BusSelector  OutputSignals=phi_theta_psi
  Bus Selector10 : BusSelector  OutputSignals=Y
  Bus Selector11 : BusSelector  OutputSignals=Z
  Bus Selector12 : BusSelector  Commented=on  OutputSignals=Xe
  Bus Selector13 : BusSelector  OutputSignals=pend_bus.phi_theta_psi
  Bus Selector14 : BusSelector  Commented=on  OutputSignals=Xe
  Bus Selector2 : BusSelector  OutputSignals=Ve
  Bus Selector3 : BusSelector  OutputSignals=DOT_phi_theta_psi
  Bus Selector4 : BusSelector  OutputSignals=Xe
  Bus Selector5 : BusSelector  OutputSignals=phi_theta_psi
  Bus Selector6 : BusSelector  OutputSignals=Ve
  Bus Selector7 : BusSelector  OutputSignals=DOT_phi_theta_psi
  Bus Selector8 : BusSelector  OutputSignals=Xe
  Bus Selector9 : BusSelector  OutputSignals=X
  Demux{,1..9} (10 alike) : Demux  Outputs=3
  EYES_ALL : Scope  NumInputPorts=12
  EYES_CMD : Scope  NumInputPorts=3
  EYES_ONE : Scope  NumInputPorts=9
  EYES_TWO : Scope  NumInputPorts=6
  From11 : From  Commented=on  GotoTag=SUT
  From13 : From  Commented=on  GotoTag=SUT
  Mux : Mux  Inputs=2
  Mux1 : Mux  Inputs=2
  Mux2 : Mux  Inputs=2
  Radians to Degrees{,1..14} (15 alike) : simulink_extras/Transformations/Radians to Degrees
  Selector : Selector  Commented=on  InputPortWidth=3  IndexOptions=Index vector (dialog)  Indices=1  OutputSizes=1
  Selector1 : Selector  Commented=on  InputPortWidth=3  IndexOptions=Index vector (dialog)  Indices=2  OutputSizes=1
  Selector2 : Selector  Commented=on  InputPortWidth=3  IndexOptions=Index vector (dialog)  Indices=1  OutputSizes=1
  Selector3 : Selector  Commented=on  InputPortWidth=3  IndexOptions=Index vector (dialog)  Indices=2  OutputSizes=1
  XY_LAGRANGE : simulink/Sinks/XY Graph  Commented=on  xmin=-1  xmax=30  ymin=-1  ymax=35  st=-1
  XY_LAGRANGE_ZOOM : simulink/Sinks/XY Graph  Commented=on  xmin=-3  xmax=3  ymin=-3  ymax=3  st=-1
  Zero-Order Hold1 : ZeroOrderHold  Commented=on  SampleTime=0.1
  Zero-Order Hold2 : ZeroOrderHold  Commented=on  SampleTime=0.1
  wires:
  SUT/1 -> [SUT]
  [SUT] -> Bus Selector/1
  Demux/2 -> EYES_ONE/2  "Ye"
  Demux/3 -> EYES_ONE/3  "Ze"
  Demux/1 -> EYES_ONE/1  "Xe"
  Bus Selector/1 -> Demux/1  "<Xe>"
  Bus Selector1/1 -> Demux1/1  "<phi_theta_psi>"
  [SUT] -> Bus Selector1/1
  Demux1/1 -> Radians to Degrees/1
  Radians to Degrees/1 -> EYES_ONE/4  "yaw_deg"
  Radians to Degrees1/1 -> EYES_ONE/5  "pitch_deg"
  Radians to Degrees2/1 -> EYES_ONE/6  "roll_deg"
  Demux1/3 -> Radians to Degrees2/1
  Demux1/2 -> Radians to Degrees1/1
  [SUT] -> Bus Selector2/1
  Demux2/2 -> EYES_TWO/2  "dot_Ye"
  Demux2/3 -> EYES_TWO/3  "dot_Ze"
  Demux2/1 -> EYES_TWO/1  "dot_Xe"
  Bus Selector2/1 -> Demux2/1  "<Ve>"
  Bus Selector3/1 -> Demux3/1  "<DOT_phi_theta_psi>"
  [SUT] -> Bus Selector3/1
  Demux3/1 -> Radians to Degrees3/1
  Radians to Degrees3/1 -> EYES_TWO/4  "dot_yaw_deg"
  Radians to Degrees4/1 -> EYES_TWO/5  "dot_pitch_deg"
  Radians to Degrees5/1 -> EYES_TWO/6  "dot_roll_deg"
  Demux3/3 -> Radians to Degrees5/1
  Demux3/2 -> Radians to Degrees4/1
  [SUT] -> Bus Selector6/1, Bus Selector4/1
  Demux4/2 -> EYES_ALL/2  "Ye"
  Demux4/3 -> EYES_ALL/3  "Ze"
  Demux4/1 -> EYES_ALL/1  "Xe"
  Bus Selector4/1 -> Demux4/1  "<Xe>"
  Bus Selector5/1 -> Demux5/1  "<phi_theta_psi>"
  [SUT] -> Bus Selector5/1
  Demux5/1 -> Radians to Degrees6/1
  Demux6/1 -> EYES_ALL/4  "Xe_dot"
  Demux6/2 -> EYES_ALL/5  "Ye_dot"
  Demux6/3 -> EYES_ALL/6  "Ze_dot"
  Demux5/3 -> Radians to Degrees8/1
  Demux5/2 -> Radians to Degrees7/1
  Bus Selector6/1 -> Demux6/1  "<Ve>"
  Radians to Degrees6/1 -> EYES_ALL/7  "yaw_deg"
  Radians to Degrees7/1 -> EYES_ALL/8  "pitch_deg"
  Radians to Degrees8/1 -> EYES_ALL/9  "roll_deg"
  Bus Selector7/1 -> Demux7/1  "<DOT_phi_theta_psi>"
  [SUT] -> Bus Selector7/1
  Demux7/1 -> Radians to Degrees9/1
  Demux7/2 -> Radians to Degrees10/1
  Demux7/3 -> Radians to Degrees11/1
  Radians to Degrees9/1 -> EYES_ALL/10  "yaw_deg_dot"
  Radians to Degrees10/1 -> EYES_ALL/11  "pitch_deg_dot"
  Radians to Degrees11/1 -> EYES_ALL/12  "roll_deg_dot"
  CMD/1 -> [CMD]
  [SUT] -> Bus Selector8/1
  Demux9/2 -> Mux1/1  "Ye"
  Demux9/1 -> Mux/1  "Xe"
  Bus Selector8/1 -> Demux9/1  "<Xe>"
  Mux/1 -> EYES_CMD/1  "X"
  Mux1/1 -> EYES_CMD/2  "Y"
  Mux2/1 -> EYES_CMD/3  "Z"
  Demux9/3 -> Mux2/1  "Ze"
  [CMD] -> Bus Selector9/1
  Bus Selector9/1 -> Mux/2  "<X>"
  [CMD] -> Bus Selector10/1
  Bus Selector10/1 -> Mux1/2  "<Y>"
  [CMD] -> Bus Selector11/1
  Bus Selector11/1 -> Mux2/2  "<Z>"
  From13/1 -> Bus Selector14/1
  Bus Selector14/1 -> Zero-Order Hold2/1  "<Xe>"
  Zero-Order Hold2/1 -> Selector1/1, Selector/1
  Selector1/1 -> XY_LAGRANGE/2
  Selector/1 -> XY_LAGRANGE/1
  [SUT] -> Bus Selector13/1
  Bus Selector13/1 -> Demux8/1  "<phi_theta_psi>"
  Demux8/3 -> Radians to Degrees14/1
  Demux8/2 -> Radians to Degrees13/1
  Demux8/1 -> Radians to Degrees12/1
  Radians to Degrees12/1 -> EYES_ONE/7  "PEND_phi"
  Radians to Degrees13/1 -> EYES_ONE/8  "PEND_theta"
  Radians to Degrees14/1 -> EYES_ONE/9  "PEND_psi"
  Zero-Order Hold1/1 -> Selector3/1, Selector2/1
  From11/1 -> Bus Selector12/1
  Selector3/1 -> XY_LAGRANGE_ZOOM/2
  Bus Selector12/1 -> Zero-Order Hold1/1  "<Xe>"
  Selector2/1 -> XY_LAGRANGE_ZOOM/1

== system bh_compare_hand_MCKG_to_Ab/Grav_FFWD ==
  In1 : Inport
  Constant3 : Constant  Value=P_veh.mass + P_pend.mass
  Gain : Gain  Gain=9.81
  Sum : Sum  Inputs=++|
  Out1 : Outport  VectorParamsAs1DForOutWhenUnconnected=off
  wires:
  Gain/1 -> Sum/1
  Constant3/1 -> Gain/1
  Sum/1 -> Out1/1
  In1/1 -> Sum/2

== system bh_compare_hand_MCKG_to_Ab/Grav_FFWD1 ==
  In1 : Inport
  Constant3 : Constant  Value=P_veh.mass + P_pend.mass
  Gain : Gain  Gain=9.81
  Sum : Sum  Inputs=++|
  Out1 : Outport  VectorParamsAs1DForOutWhenUnconnected=off
  wires:
  Gain/1 -> Sum/1
  Constant3/1 -> Gain/1
  Sum/1 -> Out1/1
  In1/1 -> Sum/2

== system bh_compare_hand_MCKG_to_Ab/Load_VEHICLE_PARAMETERS ==

== system bh_compare_hand_MCKG_to_Ab/Load_VEHICLE_PARAMETERS1 ==

== system bh_compare_hand_MCKG_to_Ab/SAR ==
  Mux : Mux  Inputs=3
  Selector : Selector  InputPortWidth=3  IndexOptions=Index vector (dialog)  Indices=[2 3 1]  OutputSizes=1
  XYZ_CMDS : Subsystem  Tag=STV Subsys  LoadFcn=sigbuilder_block('load');  StartFcn=sigbuilder_block('start');  StopFcn=sigbuilder_block('stop');  ClipboardFcn=sigbuilder_block('clipboard');  mask(Sigbuilder block){tuvar=[0:10]}
      mask help: Simulink:masks:SigbuilderBlock_MD
      mask init:
      | if ~strcmp(get_param(bdroot(gcbh),'SimulationStatus'),'stopped') tuvar = sigbuilder_block('maskInit'); end
      settings: CopyFcn=sigbuilder_block('copy');  DeleteFcn=sigbuilder_block('delete');  ModelCloseFcn=sigbuilder_block('modelClose');  PreSaveFcn=sigbuilder_block('preSave');  PauseFcn=sigbuilder_block('pause');  ContinueFcn=sigbuilder_block('continue');  NameChangeFcn=sigbuilder_block('namechange');  OpenFcn=sigbuilder_block('open',[189 32.25 551.25 400.5 ]);  CloseFcn=sigbuilder_block('close');
      mask Display: plot(0, 0, 100, 100,[2, 2, 32, 32, 2], [68, 8, 8, 68, 68],[32, 2], [38, 38], [32, 19, 2],[53, 60, 44], [32, 17, 17, 2],[16, 16, 31, 31]);txt = getActiveGroup(gcbh);text(2, 100, txt,'verticalAlignment', 'top');
  Out1 : Outport  VectorParamsAs1DForOutWhenUnconnected=off
  wires:
  XYZ_CMDS/3(Y) -> Mux/3
  XYZ_CMDS/1(Z) -> Mux/1
  XYZ_CMDS/2(X) -> Mux/2
  Mux/1 -> Selector/1
  Selector/1 -> Out1/1

== system bh_compare_hand_MCKG_to_Ab/SIGN_CONVENTIONS ==

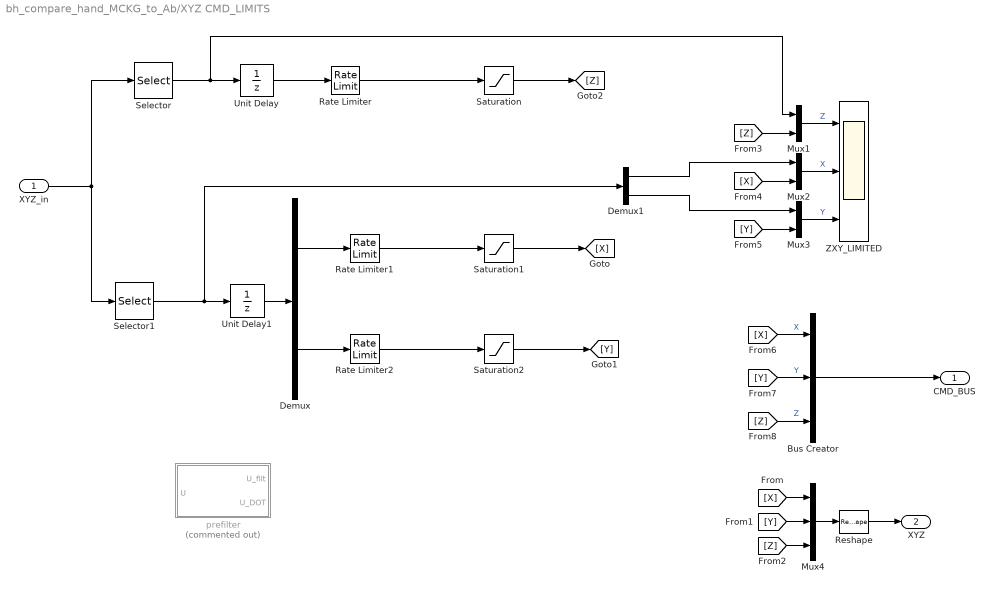
== system bh_compare_hand_MCKG_to_Ab/XYZ CMD_LIMITS ==
  XYZ_in : Inport
  Bus Creator : BusCreator  Inputs=3
  Demux : Demux  Outputs=2
  Demux1 : Demux  Outputs=2
  Mux1 : Mux  Inputs=2
  Mux2 : Mux  Inputs=2
  Mux3 : Mux  Inputs=2
  Mux4 : Mux  Inputs=3
  Rate Limiter : RateLimiter  RisingSlewLimit=2  FallingSlewLimit=-2
      settings: AttributesFormatString=|
      | Rising_rate = %<RisingSlewLimit>
      | Falling_rate = %<FallingSlewLimit>
  Rate Limiter1 : RateLimiter  RisingSlewLimit=3  FallingSlewLimit=-3
      settings: AttributesFormatString=|
      | Rising_rate = %<RisingSlewLimit>
      | Falling_rate = %<FallingSlewLimit>
  Rate Limiter2 : RateLimiter  RisingSlewLimit=3  FallingSlewLimit=-3
      settings: AttributesFormatString=|
      | Rising_rate = %<RisingSlewLimit>
      | Falling_rate = %<FallingSlewLimit>
  Reshape : Reshape  OutputDimensionality=Column vector (2-D)
  Saturation : Saturate  UpperLimit=500  LowerLimit=0
      settings: AttributesFormatString=|
      | MAX =    %<UpperLimit>
      | MIN = %<LowerLimit>
  Saturation1 : Saturate  UpperLimit=500  LowerLimit=-500
      settings: AttributesFormatString=|
      | MAX =    %<UpperLimit>
      | MIN = %<LowerLimit>
  Saturation2 : Saturate  UpperLimit=500  LowerLimit=-500
      settings: AttributesFormatString=|
      | MAX =    %<UpperLimit>
      | MIN = %<LowerLimit>
  Selector : Selector  InputPortWidth=3  IndexOptions=Index vector (dialog)  Indices=3  OutputSizes=1
  Selector1 : Selector  InputPortWidth=3  IndexOptions=Index vector (dialog)  Indices=[1 2]  OutputSizes=1
  Unit Delay : UnitDelay  SampleTime=0.01  HasFrameUpgradeWarning=on
  Unit Delay1 : UnitDelay  SampleTime=0.01  HasFrameUpgradeWarning=on
  ZXY_LIMITED : Scope  NumInputPorts=3
  prefilter : Subsystem  Commented=on  mask(Derivative Estimation){wn=2*pi*0.5, p=1}
      mask prompts: wn "Natural frequency, wn (rad/sec)"; p "Damping ratio, p"
      mask help:
      | A simple derivative estimator using a 2nd order representation between input and output.
      |
      | The integrators use a discrete FORWARd Euler rule, and a sample time needs to be specified.
      mask init:
      | str1 = sprintf('wn = %.2f', wn);
      | str2 = sprintf('p  = %.2f', p);
      | %str3 = sprintf('dt = %.2f', dt);
      | %str = char(str1,str2,str3);
      | %str3 = sprintf('dt = %.2f', dt);
      | str = char(str1,str2);
      mask Display: disp(str)
  CMD_BUS : Outport  VectorParamsAs1DForOutWhenUnconnected=off
  XYZ : Outport  Port=2  VectorParamsAs1DForOutWhenUnconnected=off
  wires:
  Selector1/1 -> Demux1/1, Unit Delay1/1
  Demux/1 -> Rate Limiter1/1
  Demux/2 -> Rate Limiter2/1
  Saturation1/1 -> [X]
  Saturation2/1 -> [Y]
  Mux4/1 -> Reshape/1
  Selector/1 -> Mux1/1, Unit Delay/1
  Rate Limiter/1 -> Saturation/1
  Unit Delay/1 -> Rate Limiter/1
  Unit Delay1/1 -> Demux/1
  Rate Limiter1/1 -> Saturation1/1
  Rate Limiter2/1 -> Saturation2/1
  [X] -> Mux4/1
  [Y] -> Mux4/2
  [Z] -> Mux4/3
  Saturation/1 -> [Z]
  [Z] -> Mux1/2
  [Y] -> Mux3/2
  Demux1/1 -> Mux2/1
  Demux1/2 -> Mux3/1
  [X] -> Mux2/2
  Mux1/1 -> ZXY_LIMITED/1  "Z"
  Mux2/1 -> ZXY_LIMITED/2  "X"
  Mux3/1 -> ZXY_LIMITED/3  "Y"
  Bus Creator/1 -> CMD_BUS/1
  [Y] -> Bus Creator/2  "Y"
  [X] -> Bus Creator/1  "X"
  [Z] -> Bus Creator/3  "Z"
  Reshape/1 -> XYZ/1
  XYZ_in/1 -> Selector1/1, Selector/1

== system bh_compare_hand_MCKG_to_Ab/a_circle1 ==
  Clock : Clock
  Clock1 : Clock
  Constant4 : Constant  Value=0  VectorParams1D=off
  Constant5 : Constant  Value=20  VectorParams1D=off
  Constant6 : Constant  Value=2  VectorParams1D=off
  Constant7 : Constant  VectorParams1D=off
  Constant8 : Constant  Value=0.05  VectorParams1D=off
  MATLAB Function : MATLAB Function  TreatAsAtomicUnit=on
  Mux1 : Mux  Inputs=3
  Reshape1 : Reshape  OutputDimensionality=Column vector (2-D)
  Reshape2 : Reshape  OutputDimensionality=Column vector (2-D)
  Signal Builder : Subsystem  Tag=STV Subsys  LoadFcn=sigbuilder_block('load');  StartFcn=sigbuilder_block('start');  StopFcn=sigbuilder_block('stop');  ClipboardFcn=sigbuilder_block('clipboard');  mask(Sigbuilder block){tuvar=[0:10]}
      mask help: Simulink:masks:SigbuilderBlock_MD
      mask init:
      | if ~strcmp(get_param(bdroot(gcbh),'SimulationStatus'),'stopped') tuvar = sigbuilder_block('maskInit'); end
      settings: CopyFcn=sigbuilder_block('copy');  DeleteFcn=sigbuilder_block('delete');  ModelCloseFcn=sigbuilder_block('modelClose');  PreSaveFcn=sigbuilder_block('preSave');  PauseFcn=sigbuilder_block('pause');  ContinueFcn=sigbuilder_block('continue');  NameChangeFcn=sigbuilder_block('namechange');  OpenFcn=sigbuilder_block('open',[437.6 199.2 550.4 400 ]);  CloseFcn=sigbuilder_block('close');
      mask Display: plot(0, 0, 100, 100,[2, 2, 32, 32, 2], [68, 8, 8, 68, 68],[32, 2], [38, 38], [32, 19, 2],[53, 60, 44], [32, 17, 17, 2],[16, 16, 31, 31]);txt = getActiveGroup(gcbh);text(2, 100, txt,'verticalAlignment', 'top');
  Subsystem : Subsystem
  Switch : Switch  Criteria=u2 > Threshold  Threshold=20
  Out1 : Outport  VectorParamsAs1DForOutWhenUnconnected=off
  wires:
  Switch/1 -> Out1/1
  MATLAB Function/1(XYZ) -> Reshape2/1
  Constant6/1 -> MATLAB Function/3(RADIUS)
  Constant7/1 -> MATLAB Function/4(ztgt)
  Subsystem/1(w_rad_psec) -> MATLAB Function/5(w)
  Constant5/1 -> MATLAB Function/2(t_to_start)
  Reshape1/1 -> Switch/3
  Constant4/1 -> Mux1/2
  Signal Builder/1(Signal 1) -> Mux1/1
  Signal Builder/2(Signal 2) -> Mux1/3
  Mux1/1 -> Reshape1/1
  Clock/1 -> Switch/2
  Clock1/1 -> MATLAB Function/1(t_clock)
  Constant8/1 -> Subsystem/1(RPS)
  Reshape2/1 -> Switch/1

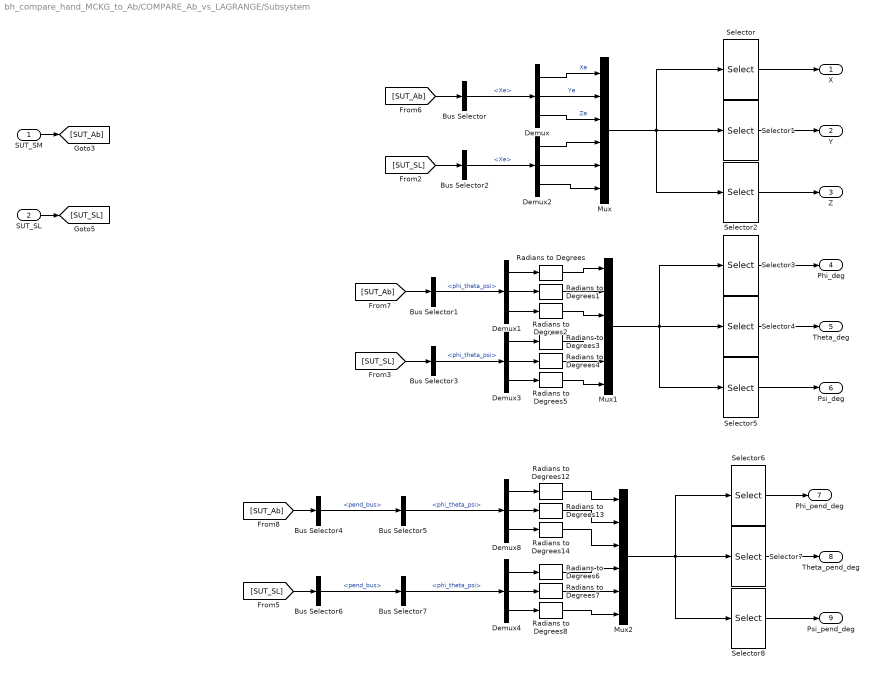
== system bh_compare_hand_MCKG_to_Ab/COMPARE_Ab_vs_LAGRANGE/Subsystem ==
  SUT_SM : Inport
  SUT_SL : Inport  Port=2
  Bus Selector : BusSelector  OutputSignals=Xe
  Bus Selector{1,3,5,7} (4 alike) : BusSelector  OutputSignals=phi_theta_psi
  Bus Selector2 : BusSelector  OutputSignals=Xe
  Bus Selector4 : BusSelector  OutputSignals=pend_bus
  Bus Selector6 : BusSelector  OutputSignals=pend_bus
  Demux{,1..4,8} (6 alike) : Demux  Outputs=3
  Mux : Mux  Inputs=6
  Mux1 : Mux  Inputs=6
  Mux2 : Mux  Inputs=6
  Radians to Degrees{,1..8,12..14} (12 alike) : simulink_extras/Transformations/Radians to Degrees
  Selector : Selector  InputPortWidth=6  IndexOptions=Index vector (dialog)  Indices=[1 4]  OutputSizes=1
  Selector1 : Selector  InputPortWidth=6  IndexOptions=Index vector (dialog)  Indices=[2 5]  OutputSizes=1
  Selector2 : Selector  InputPortWidth=6  IndexOptions=Index vector (dialog)  Indices=[3 6]  OutputSizes=1
  Selector3 : Selector  InputPortWidth=6  IndexOptions=Index vector (dialog)  Indices=[1 4]  OutputSizes=1
  Selector4 : Selector  InputPortWidth=6  IndexOptions=Index vector (dialog)  Indices=[2 5]  OutputSizes=1
  Selector5 : Selector  InputPortWidth=6  IndexOptions=Index vector (dialog)  Indices=[3 6]  OutputSizes=1
  Selector6 : Selector  InputPortWidth=6  IndexOptions=Index vector (dialog)  Indices=[1 4]  OutputSizes=1
  Selector7 : Selector  InputPortWidth=6  IndexOptions=Index vector (dialog)  Indices=[2 5]  OutputSizes=1
  Selector8 : Selector  InputPortWidth=6  IndexOptions=Index vector (dialog)  Indices=[3 6]  OutputSizes=1
  X : Outport  VectorParamsAs1DForOutWhenUnconnected=off
  Y : Outport  Port=2  VectorParamsAs1DForOutWhenUnconnected=off
  Z : Outport  Port=3  VectorParamsAs1DForOutWhenUnconnected=off
  Phi_deg : Outport  Port=4  VectorParamsAs1DForOutWhenUnconnected=off
  Theta_deg : Outport  Port=5  VectorParamsAs1DForOutWhenUnconnected=off
  Psi_deg : Outport  Port=6  VectorParamsAs1DForOutWhenUnconnected=off
  Phi_pend_deg : Outport  Port=7  VectorParamsAs1DForOutWhenUnconnected=off
  Theta_pend_deg : Outport  Port=8  VectorParamsAs1DForOutWhenUnconnected=off
  Psi_pend_deg : Outport  Port=9  VectorParamsAs1DForOutWhenUnconnected=off
  wires:
  SUT_SL/1 -> [SUT_SL]
  SUT_SM/1 -> [SUT_Ab]
  Demux8/2 -> Radians to Degrees13/1
  [SUT_Ab] -> Bus Selector1/1
  Bus Selector1/1 -> Demux1/1  "<phi_theta_psi>"
  Bus Selector/1 -> Demux/1  "<Xe>"
  Demux1/2 -> Radians to Degrees1/1
  Demux8/3 -> Radians to Degrees14/1
  [SUT_Ab] -> Bus Selector4/1
  Demux8/1 -> Radians to Degrees12/1
  [SUT_Ab] -> Bus Selector/1
  Demux1/1 -> Radians to Degrees/1
  Demux1/3 -> Radians to Degrees2/1
  [SUT_SL] -> Bus Selector2/1
  Bus Selector2/1 -> Demux2/1  "<Xe>"
  Demux3/1 -> Radians to Degrees3/1
  [SUT_SL] -> Bus Selector3/1
  Bus Selector3/1 -> Demux3/1  "<phi_theta_psi>"
  Demux3/2 -> Radians to Degrees4/1
  Demux3/3 -> Radians to Degrees5/1
  Bus Selector4/1 -> Bus Selector5/1  "<pend_bus>"
  Bus Selector5/1 -> Demux8/1  "<phi_theta_psi>"
  [SUT_SL] -> Bus Selector6/1
  Demux4/2 -> Radians to Degrees7/1
  Demux4/1 -> Radians to Degrees6/1
  Demux4/3 -> Radians to Degrees8/1
  Bus Selector6/1 -> Bus Selector7/1  "<pend_bus>"
  Bus Selector7/1 -> Demux4/1  "<phi_theta_psi>"
  Demux2/2 -> Mux/5
  Demux2/3 -> Mux/6
  Demux2/1 -> Mux/4
  Demux/3 -> Mux/3  "Ze"
  Demux/2 -> Mux/2  "Ye"
  Demux/1 -> Mux/1  "Xe"
  Radians to Degrees5/1 -> Mux1/6
  Radians to Degrees4/1 -> Mux1/5
  Radians to Degrees3/1 -> Mux1/4
  Radians to Degrees2/1 -> Mux1/3
  Radians to Degrees1/1 -> Mux1/2
  Radians to Degrees/1 -> Mux1/1
  Radians to Degrees12/1 -> Mux2/1
  Radians to Degrees13/1 -> Mux2/2
  Radians to Degrees14/1 -> Mux2/3
  Radians to Degrees6/1 -> Mux2/4
  Radians to Degrees7/1 -> Mux2/5
  Radians to Degrees8/1 -> Mux2/6
  Mux2/1 -> Selector8/1, Selector6/1, Selector7/1
  Mux/1 -> Selector/1, Selector2/1, Selector1/1
  Mux1/1 -> Selector5/1, Selector3/1, Selector4/1
  Selector2/1 -> Z/1
  Selector1/1 -> Y/1
  Selector/1 -> X/1
  Selector5/1 -> Psi_deg/1
  Selector4/1 -> Theta_deg/1
  Selector3/1 -> Phi_deg/1
  Selector6/1 -> Phi_pend_deg/1
  Selector8/1 -> Psi_pend_deg/1
  Selector7/1 -> Theta_pend_deg/1

== system bh_compare_hand_MCKG_to_Ab/CONT_SYS W_MOT_CMDS1/MOTOR_sys ==
  w_CMD : Inport
  Demux : Demux
  MOTOR_1 : Subsystem
      mask Display: image('bh_PIC_MOTOR.jpg');
  MOTOR_2 : Subsystem
      mask Display: image('bh_PIC_MOTOR.jpg');
  MOTOR_3 : Subsystem
      mask Display: image('bh_PIC_MOTOR.jpg');
  MOTOR_4 : Subsystem
      mask Display: image('bh_PIC_MOTOR.jpg');
  Mux : Mux
  w CMD vs Actual : Scope  NumInputPorts=4
  w_MUX : Subsystem
  w : Outport  VectorParamsAs1DForOutWhenUnconnected=off
  wires:
  MOTOR_4/1(w) -> Mux/4
  MOTOR_3/1(w) -> Mux/3
  MOTOR_2/1(w) -> Mux/2
  MOTOR_1/1(w) -> Mux/1
  Demux/1 -> MOTOR_1/1(w_CMD)
  Demux/2 -> MOTOR_2/1(w_CMD)
  Demux/3 -> MOTOR_3/1(w_CMD)
  Demux/4 -> MOTOR_4/1(w_CMD)
  w_CMD/1 -> [W_CMD], Demux/1
  w_MUX/4(w4) -> w CMD vs Actual/4
  w_MUX/2(w2) -> w CMD vs Actual/2
  w_MUX/3(w3) -> w CMD vs Actual/3
  w_MUX/1(w1) -> w CMD vs Actual/1
  [W_CMD] -> w_MUX/1(W_CMD)
  Mux/1 -> w_MUX/2(W), w/1

== system bh_compare_hand_MCKG_to_Ab/CONT_SYS W_MOT_CMDS1/SIGN_CONVENTIONS ==

== system bh_compare_hand_MCKG_to_Ab/CONT_SYS W_MOT_CMDS1/W2_checker ==
  w2_CMD : Inport
  Assertion{,1..3} (4 alike) : Assertion
  Compare To Constant : simulink/Logic and Bit Operations/Compare To Constant  relop=>=  const=0  OutDataTypeStr=boolean
  Demux : Demux
  w2 : Outport  VectorParamsAs1DForOutWhenUnconnected=off
  wires:
  w2_CMD/1 -> w2/1, Compare To Constant/1
  Compare To Constant/1 -> Demux/1
  Demux/1 -> Assertion/1
  Demux/4 -> Assertion3/1
  Demux/3 -> Assertion2/1
  Demux/2 -> Assertion1/1

== system bh_compare_hand_MCKG_to_Ab/CONT_SYS W_MOT_CMDS2/MOTOR_sys ==
  w_CMD : Inport
  Demux : Demux
  MOTOR_1 : Subsystem
      mask Display: image('bh_PIC_MOTOR.jpg');
  MOTOR_2 : Subsystem
      mask Display: image('bh_PIC_MOTOR.jpg');
  MOTOR_3 : Subsystem
      mask Display: image('bh_PIC_MOTOR.jpg');
  MOTOR_4 : Subsystem
      mask Display: image('bh_PIC_MOTOR.jpg');
  Mux : Mux
  w CMD vs Actual : Scope  NumInputPorts=4
  w_MUX : Subsystem
  w : Outport  VectorParamsAs1DForOutWhenUnconnected=off
  wires:
  MOTOR_4/1(w) -> Mux/4
  MOTOR_3/1(w) -> Mux/3
  MOTOR_2/1(w) -> Mux/2
  MOTOR_1/1(w) -> Mux/1
  Demux/1 -> MOTOR_1/1(w_CMD)
  Demux/2 -> MOTOR_2/1(w_CMD)
  Demux/3 -> MOTOR_3/1(w_CMD)
  Demux/4 -> MOTOR_4/1(w_CMD)
  w_CMD/1 -> [W_CMD], Demux/1
  w_MUX/4(w4) -> w CMD vs Actual/4
  w_MUX/2(w2) -> w CMD vs Actual/2
  w_MUX/3(w3) -> w CMD vs Actual/3
  w_MUX/1(w1) -> w CMD vs Actual/1
  [W_CMD] -> w_MUX/1(W_CMD)
  Mux/1 -> w_MUX/2(W), w/1

== system bh_compare_hand_MCKG_to_Ab/CONT_SYS W_MOT_CMDS2/SIGN_CONVENTIONS ==

== system bh_compare_hand_MCKG_to_Ab/CONT_SYS W_MOT_CMDS2/W2_checker ==
  w2_CMD : Inport
  Assertion{,1..3} (4 alike) : Assertion
  Compare To Constant : simulink/Logic and Bit Operations/Compare To Constant  relop=>=  const=0  OutDataTypeStr=boolean
  Demux : Demux
  w2 : Outport  VectorParamsAs1DForOutWhenUnconnected=off
  wires:
  w2_CMD/1 -> w2/1, Compare To Constant/1
  Compare To Constant/1 -> Demux/1
  Demux/1 -> Assertion/1
  Demux/4 -> Assertion3/1
  Demux/3 -> Assertion2/1
  Demux/2 -> Assertion1/1

== system bh_compare_hand_MCKG_to_Ab/SAR/XYZ_CMDS ==
  Demux : Demux  Tag=STV Demux  Outputs=3
      settings: DisplayOption=none
  FromWs : FromWorkspace  Tag=STV FromWs  VariableName=tuvar
      SigBuilderData=|
      | common.afterFinalStr = 'Extrapolate'
      | common.sampleTime = 0
      | dataSet(1).timeRange = [0 200]
      | dataSet(1).name = 'small_steps'
      | dataSet(2).timeRange = [0 200]
      | dataSet(2).name = 'zStairs_xyConstVEL'
      | dataSet(3).timeRange = [0 500]
      | dataSet(3).name = 'sineWaves'
      | dataSet(4).timeRange = [0 200]
      | dataSet(4).name = 'ZERO'
      | dataSet(5).timeRange = [0 200]
      | dataSet(5).name = 'SEARCH_P1'
      | sbobj.Name = 'Signal Builder'
      | sbobj.Groups(1).Name = 'small_steps'
      | sbobj.Groups(1).Signals(1).Name = 'Z'
      | sbobj.Groups(1).Signals(1).XData = [0 10 10.000001 20 20.000001 30 30.000001 55 200]
      | sbobj.Groups(1).Signals(1).YData = [0 0 2 2 2 2 2 2 2]
      | sbobj.Groups(1).Signals(2).Name = 'X'
      | sbobj.Groups(1).Signals(2).XData = [0 10 10.000001 20 20.000001 30 30.000001 55 200]
      | sbobj.Groups(1).Signals(2).YData = [0 0 0 0 3 3 3 3 3]
      | sbobj.Groups(1).Signals(3).Name = 'Y'
      | sbobj.Groups(1).Signals(3).XData = [0 10 10.000001 20 20.000001 30 30.000001 55 200]
      | sbobj.Groups(1).Signals(3).YData = [0 0 0 0 0 0 1 1 1]
      | sbobj.Groups(1).TimeRange = [0 200]
      | sbobj.Groups(2).Name = 'zStairs_xyConstVEL'
      | sbobj.Groups(2).Signals(1).Name = 'Z'
      | sbobj.Groups(2).Signals(1).XData = [0 10 10.000001 20 20.000001 30 30.000001 40 40.000001 55 200]
      | sbobj.Groups(2).Signals(1).YData = [0 0 1 1 2 2 1 1 0 0 0]
      | sbobj.Groups(2).Signals(2).Name = 'X'
      | sbobj.Groups(2).Signals(2).XData = [0 10 10.000001 20 20.000001 30 30.000001 40 40.000001 55 200]
      | sbobj.Groups(2).Signals(2).YData = [0 1 1.0000001 2 2.0000001 3 3.0000001 4 4.0000001 5.5 20]
      | sbobj.Groups(2).Signals(3).Name = 'Y'
      | sbobj.Groups(2).Signals(3).XData = [0 10 10.000001 20 20.000001 30 30.000001 40 40.000001 55 200]
      | sbobj.Groups(2).Signals(3).YData = [0 0.5 0.50000005 1 1.00000005 1.5 1.50000005 2 2.00000005 2.75 10]
      | sbobj.Groups(2).TimeRange = [0 200]
      | sbobj.Groups(3).Name = 'sineWaves'
      | sbobj.Groups(3).Signals(1).Name = 'Z'
      | sbobj.Groups(3).Signals(1).XData = [0 0.1 0.2 0.3 0.4 0.5 0.6 0.7 0.8 0.9 1 1.1 ... (5001 elements, 1x5001)]
      | sbobj.Groups(3).Signals(1).YData = [0 0.0314107325553 0.0627904665622 0.0941082340641 0.125333128258 0.156434333994 0.18738115819 0.218143060119 0.248689681547 0.278990876699 0.309016742004 0.338737645607 ... (5001 elements, 1x5001)]
      | sbobj.Groups(3).Signals(2).Name = 'X'
      | sbobj.Groups(3).Signals(2).XData = [0 0.1 0.2 0.3 0.4 0.5 0.6 0.7 0.8 0.9 1 1.1 ... (5001 elements, 1x5001)]
      | sbobj.Groups(3).Signals(2).YData = [0 0.01 0.02 0.03 0.04 0.05 0.06 0.07 0.08 0.09 0.1 0.11 ... (5001 elements, 1x5001)]
      | sbobj.Groups(3).Signals(3).Name = 'Y'
      | sbobj.Groups(3).Signals(3).XData = [0 0.1 0.2 0.3 0.4 0.5 0.6 0.7 0.8 0.9 1 1.1 ... (5001 elements, 1x5001)]
      | sbobj.Groups(3).Signals(3).YData = [0 0.0157073040455 0.0314107325553 0.04710641095 0.0627904665622 0.0784590295926 0.0941082340641 0.109734218776 0.125333128258 0.140901113717 0.156434333994 0.171928956505 ... (5001 elements, 1x5001)]
      | sbobj.Groups(3).TimeRange = [0 500]
      | sbobj.Groups(4).Name = 'ZERO'
      | sbobj.Groups(4).Signals(1).Name = 'Z'
      | sbobj.Groups(4).Signals(1).XData = [0 200]
      | sbobj.Groups(4).Signals(1).YData = [0 0]
      | sbobj.Groups(4).Signals(2).Name = 'X'
      | sbobj.Groups(4).Signals(2).XData = [0 200]
      | sbobj.Groups(4).Signals(2).YData = [0 0]
      | sbobj.Groups(4).Signals(3).Name = 'Y'
      | sbobj.Groups(4).Signals(3).XData = [0 200]
      | sbobj.Groups(4).Signals(3).YData = [0 0]
      | sbobj.Groups(4).TimeRange = [0 200]
      | sbobj.Groups(5).Name = 'SEARCH_P1'
      | sbobj.Groups(5).Signals(1).Name = 'Z'
      | sbobj.Groups(5).Signals(1).XData = [0 7 27 32 52 57 77 82 102 107 127 132 157 187 200]
      | sbobj.Groups(5).Signals(1).YData = [0 5 5 5 5 5 5 5 5 5 5 5 5 0 0]
      | sbobj.Groups(5).Signals(2).Name = 'X'
      | sbobj.Groups(5).Signals(2).XData = [0 7 27 32 52 57 77 82 102 107 127 132 157 187 200]
      | sbobj.Groups(5).Signals(2).YData = [0 5 25 25 5 5 25 25 5 5 25 25 0 0 0]
      | sbobj.Groups(5).Signals(3).Name = 'Y'
      | sbobj.Groups(5).Signals(3).XData = [0 7 27 32 52 57 77 82 102 107 127 132 157 187 200]
      | sbobj.Groups(5).Signals(3).YData = [0 5 5 10 10 15 15 20 20 25 25 30 30 0 0]
      | sbobj.Groups(5).TimeRange = [0 200]
  Z : Outport  VectorParamsAs1DForOutWhenUnconnected=off
  X : Outport  Tag=STV Outport  Port=2  VectorParamsAs1DForOutWhenUnconnected=off
  Y : Outport  Tag=STV Outport  Port=3  VectorParamsAs1DForOutWhenUnconnected=off
  wires:
  Demux/1 -> Z/1
  FromWs/1 -> Demux/1
  Demux/2 -> X/1
  Demux/3 -> Y/1
